simulink model "Punto_4"  (R2021a)
settings: Solver=VariableStepAuto  StartTime=0.0  StopTime=25  RelTol=1e-3
values from neighbouring files (symbols this model uses):
  K = Ka(1:order(P))    [Problema_3.m]
  kI = -Ka(end)    [Problema_3.m]
  u0 = 1    [Problema_3.m]
  x0 = [2, 1, 1]    [Problema_3.m]
  y0 = 1    [Problema_3.m]
settings Model: Creator=Santiago  LastModifiedBy=Santiago

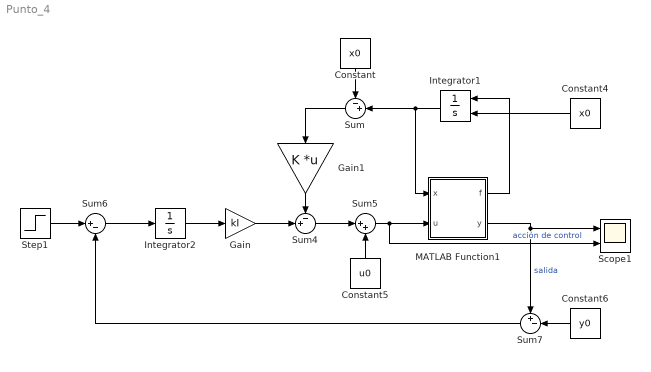
== system Punto_4 ==
  Constant : Constant  Value=x0
  Constant4 : Constant  Value=x0
  Constant5 : Constant  Value=u0
  Constant6 : Constant  Value=y0
  Gain : Gain  Gain=kI
  Gain1 : Gain  Gain=K  Multiplication=Matrix(K*u) (u vector)
  Integrator1 : Integrator  InitialConditionSource=external
  Integrator2 : Integrator
  MATLAB Function1 : MATLAB Function  TreatAsAtomicUnit=on
  Scope1 : Scope  NumInputPorts=2
  Step1 : Step  After=0.1  SampleTime=0
  Sum : Sum  Inputs=-+|
  Sum4 : Sum  Inputs=-+|
  Sum5 : Sum  Inputs=|++
  Sum6 : Sum  Inputs=|+-
  Sum7 : Sum  Inputs=+-|
  wires:
  Integrator1/1 -> Sum/2, MATLAB Function1/1(x)
  Integrator2/1 -> Gain/1
  Constant4/1 -> Integrator1/2
  Sum6/1 -> Integrator2/1
  Constant6/1 -> Sum7/2
  Gain/1 -> Sum4/2
  MATLAB Function1/2(y) -> Sum7/1, Scope1/1  "salida"
  Sum7/1 -> Sum6/2
  Sum5/1 -> Scope1/2, MATLAB Function1/2(u)  "acción de control"
  Constant5/1 -> Sum5/2
  MATLAB Function1/1(f) -> Integrator1/1
  Gain1/1 -> Sum4/1
  Step1/1 -> Sum6/1
  Sum4/1 -> Sum5/1
  Sum/1 -> Gain1/1
  Constant/1 -> Sum/1

== matlab function Punto_4/MATLAB Function1 ==
  data: x input; u input; f output; y output
function [f,y] = fcn(x,u)

p = 0.02;
f1 = (-sqrt(x(1) - x(2)) + x(3) )/x(1)^2;
f2 = (sqrt( x(1) - x(2) ) - sqrt( x(2)) )/x(2)^2;
f3 = -p * x(3) + p * u;
f=[f1; f2; f3];

y=x(2);
